simulink model "BlockDiagram"  (R2015b)
settings: Solver=VariableStepAuto  StartTime=0.0  StopTime=10.0  RelTol=1e-3
undefined symbols (not defined in the file): kd, kf, ki, kp
settings Model: Creator=aj  LastModifiedBy=aj

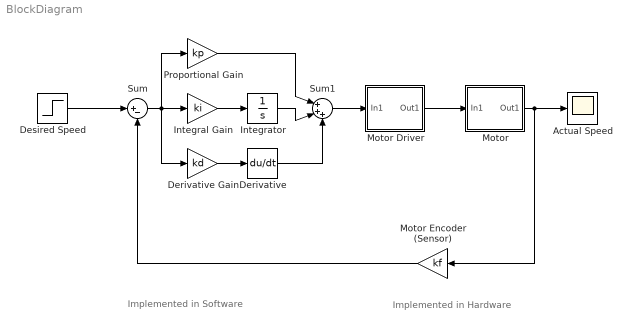
== system BlockDiagram ==
  note: Implemented in Hardware
  note: Implemented in Software
  Actual Speed : Scope
  Derivative : Derivative
  Derivative Gain : Gain  Gain=kd
  Desired Speed : Step  SampleTime=0
  Integral Gain : Gain  Gain=ki
  Integrator : Integrator
  Motor : Subsystem
  Motor Driver : Subsystem
  Motor Encoder (Sensor) : Gain  Gain=kf
  Proportional Gain : Gain  Gain=kp
  Sum : Sum  Inputs=|+-
  Sum1 : Sum  Inputs=|+++
  wires:
  Desired Speed/1 -> Sum/1
  Sum/1 -> Proportional Gain/1, Derivative Gain/1, Integral Gain/1
  Motor Encoder (Sensor)/1 -> Sum/2
  Integral Gain/1 -> Integrator/1
  Derivative Gain/1 -> Derivative/1
  Proportional Gain/1 -> Sum1/1
  Integrator/1 -> Sum1/2
  Derivative/1 -> Sum1/3
  Sum1/1 -> Motor Driver/1(In1)
  Motor Driver/1(Out1) -> Motor/1(In1)
  Motor/1(Out1) -> Actual Speed/1, Motor Encoder (Sensor)/1

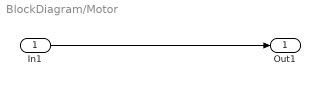
== system BlockDiagram/Motor ==
  In1 : Inport
  Out1 : Outport
  wires:
  In1/1 -> Out1/1

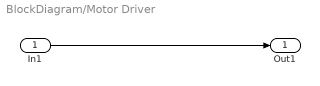
== system BlockDiagram/Motor Driver ==
  In1 : Inport
  Out1 : Outport
  wires:
  In1/1 -> Out1/1
